simulink model "bh_dewarp_test"  (R2017a)
settings: Solver=FixedStepDiscrete  StartTime=0.0  StopTime=15  RelTol=1e-3
PreLoadFcn:
  | bh_create_cv_neareset_BUS_OBJ_for_simulink()
  | fprintf('\n\n### just did a preload TASK !');
undefined symbols (not defined in the file or in its folder): gray
libraries: dspvision x1, visiongeotforms x1
settings Model: FPTRunName=Active  ExtModeAutoUpdateStatusClock=off  Creator=The MathWorks, Inc.  LastModifiedBy=bhorton
settings DataIOCC: LimitDataPoints=on  SaveFormat=Array  SaveOutput=off  SaveTime=off  SignalLoggingName=sigsOut
settings OptimizationCC: ExpressionDepthLimit=2147483647  InitFltsAndDblsToZero=on  LifeSpan=inf  BufferReusableBoundary=off
settings DebuggingCC: SaveWithParameterizedLinksMsg=none  UnderspecifiedInitializationDetection=Classic  MergeDetectMultiDrivingBlocksExec=none  CheckExecutionContextPreStartOutputMsg=on  CheckExecutionContextRuntimeOutputMsg=on  SignalResolutionControl=TryResolveAllWithWarning  MultiTaskDSMMsg=warning  MultiTaskCondExecSysMsg=none  ParameterPrecisionLossMsg=none  FcnCallInpInsideContextMsg=warning  BusObjectLabelMismatch=none  StateNameClashWarn=warning  StrictBusMsg=None  SFUnexpectedBacktrackingDiag=warning  SFNoUnconditionalDefaultTransitionDiag=warning  SFExecutionAtInitializationDiag=none
settings HardwareCC: ProdBitPerPointer=32  ProdBitPerSizeT=32  ProdBitPerPtrDiffT=32  ProdLargestAtomicFloat=None  ProdIntDivRoundTo=Undefined  ProdEndianess=Unspecified  ProdWordSize=32  ProdHWDeviceType=32-bit Generic  TargetBitPerPointer=64  TargetBitPerSizeT=64  TargetBitPerPtrDiffT=64  TargetLongLongMode=on  TargetIntDivRoundTo=Zero  TargetEndianess=LittleEndian  TargetWordSize=64  TargetHWDeviceType=Generic->MATLAB Host Computer  ProdEqTarget=off
settings ModelReferenceCC: PropagateSignalLabelsOutOfModel=off
settings GRTTargetCC: TargetFcnLib=ansi_tfl_tmw.mat  TargetLangStandard=C89/C90 (ANSI)  GeneratePreprocessorConditionals=Disable all  CombineOutputUpdateFcns=off  GRTInterface=on
settings ConfigComp: CovMetricSettings=dw  CovHtmlReporting=on  CovSaveCumulativeToWorkspaceVar=on  CovSaveSingleToWorkspaceVar=on  CovExternalEMLEnable=off

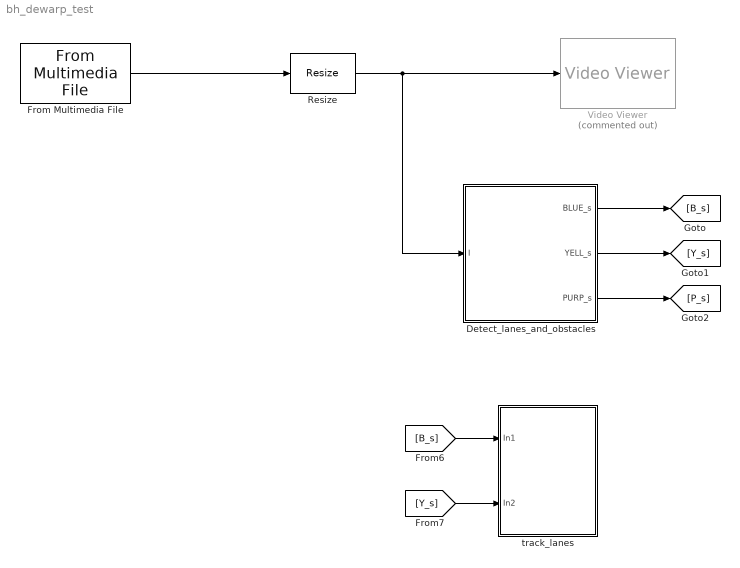
== system bh_dewarp_test ==
  Detect_lanes_and_obstacles : Subsystem
  From Multimedia File : dspvision/From Multimedia File  inputFilename=C:\bh\users_EV\Competitions\QUT_Droid_Racing_Challenge\DEMOS\sandpit\bh_vis_for_CODEGEN\TEST_VIDEO_FOR_SL_240x320.avi  loop=on  numPlays=1  outputStreams=Video only  videoDataType=uint8  audioDataType=int16  inheritSampleTime=on  userDefinedSampleTime=1/30  noAudioOutput=off  isIntensityVideo=off  fourcc=RGB  colorVideoFormat=One multidimensional signal  outputEOF=off  dataOrg=Column-major  audioFrameSize=1024  computeAudioFrameSize=off  outSamplingMode=Frame based
      settings: SourceProductBaseCode=VP
  Resize : visiongeotforms/Resize  specify=Number of output rows and columns  rfactor=[180 240]  outCols=25  outRows=25  outRowsCols=[180 240]  interp_method=Bilinear  antialias=off  useROI=off  roiFlag=off  prodOutputMode=Binary point scaling  prodOutputWordLength=32  prodOutputFracLength=10  roundingMode=Nearest  overflowMode=on
      settings: SourceProductName=Computer Vision System Toolbox  SourceProductBaseCode=VP
  Video Viewer : VideoViewer  Commented=on  colormapValue=gray(256)  FigPos=[2034 1219 418 304]
  track_lanes : Subsystem
  wires:
  From Multimedia File/1 -> Resize/1
  Detect_lanes_and_obstacles/1(BLUE_s) -> [B_s]
  Detect_lanes_and_obstacles/2(YELL_s) -> [Y_s]
  Detect_lanes_and_obstacles/3(PURP_s) -> [P_s]
  [B_s] -> track_lanes/1(In1)
  Resize/1 -> Detect_lanes_and_obstacles/1(I), Video Viewer/1
  [Y_s] -> track_lanes/2(In2)

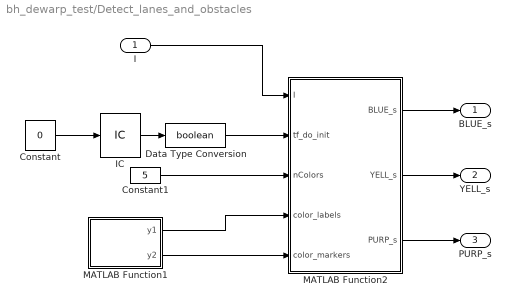
== system bh_dewarp_test/Detect_lanes_and_obstacles ==
  I : Inport
  Constant : Constant  Value=0  OutDataTypeStr=boolean
  Constant1 : Constant  Value=5  OutDataTypeStr=double
  Data Type Conversion : DataTypeConversion  OutDataTypeStr=boolean
  IC : InitialCondition
  MATLAB Function1 : MATLAB Function  TreatAsAtomicUnit=on
  MATLAB Function2 : MATLAB Function  TreatAsAtomicUnit=on
  BLUE_s : Outport
  YELL_s : Outport  Port=2
  PURP_s : Outport  Port=3
  wires:
  Constant/1 -> IC/1
  Data Type Conversion/1 -> MATLAB Function2/2(tf_do_init)
  IC/1 -> Data Type Conversion/1
  Constant1/1 -> MATLAB Function2/3(nColors)
  MATLAB Function1/1(y1) -> MATLAB Function2/4(color_labels)
  MATLAB Function1/2(y2) -> MATLAB Function2/5(color_markers)
  I/1 -> MATLAB Function2/1(I)
  MATLAB Function2/3(PURP_s) -> PURP_s/1
  MATLAB Function2/2(YELL_s) -> YELL_s/1
  MATLAB Function2/1(BLUE_s) -> BLUE_s/1

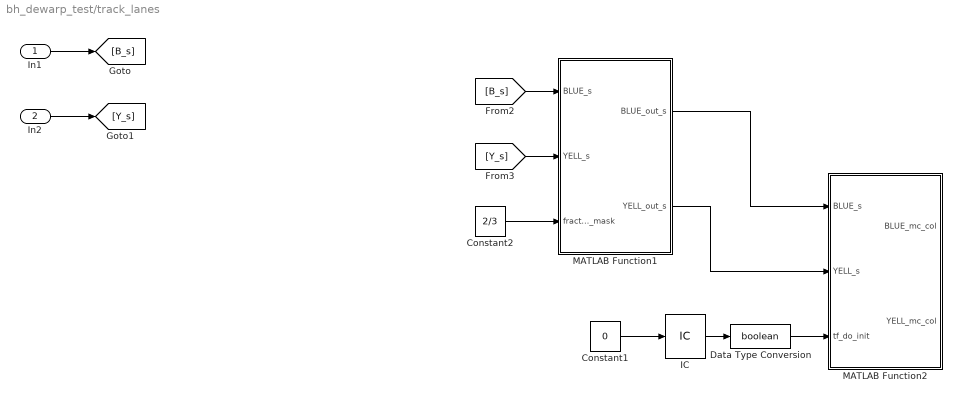
== system bh_dewarp_test/track_lanes ==
  In1 : Inport
  In2 : Inport  Port=2
  Constant1 : Constant  Value=0  OutDataTypeStr=boolean
  Constant2 : Constant  Value=2/3  OutDataTypeStr=double
  Data Type Conversion : DataTypeConversion  OutDataTypeStr=boolean
  IC : InitialCondition
  MATLAB Function1 : MATLAB Function  TreatAsAtomicUnit=on
  MATLAB Function2 : MATLAB Function  TreatAsAtomicUnit=on
  wires:
  In2/1 -> [Y_s]
  In1/1 -> [B_s]
  IC/1 -> Data Type Conversion/1
  Constant1/1 -> IC/1
  Data Type Conversion/1 -> MATLAB Function2/3(tf_do_init)
  MATLAB Function1/2(YELL_out_s) -> MATLAB Function2/2(YELL_s)
  MATLAB Function1/1(BLUE_out_s) -> MATLAB Function2/1(BLUE_s)
  [Y_s] -> MATLAB Function1/2(YELL_s)
  [B_s] -> MATLAB Function1/1(BLUE_s)
  Constant2/1 -> MATLAB Function1/3(fract_for_top_mask)

== matlab function bh_dewarp_test/Detect_lanes_and_obstacles/MATLAB Function1 ==
  data: y1 output; y2 output
function [y1, y2] = fcn()

y1 = [0,1,2,3,4];

y2 = [ ...
       -7.8436  -30.0394;
      -10.2908   36.4110;
       42.5297   -8.7231;
        2.1904    1.6907;
        4.0686    3.2113;
        ];
    
end

== matlab function bh_dewarp_test/track_lanes/MATLAB Function1 ==
  data: BLUE_s input Bus: lane_info_BUS; YELL_s input Bus: lane_info_BUS; fract_for_top_mask input; BLUE_out_s output Bus: lane_info_BUS; YELL_out_s output Bus: lane_info_BUS
function [BLUE_out_s, YELL_out_s] = ...
     pre_process_lanes(BLUE_s, YELL_s, fract_for_top_mask) %#codegen

coder.extrinsic('bh_my_lane_preprocess_mask')

[BLUE_out_s, YELL_out_s] = ...
    bh_my_lane_preprocess_mask(BLUE_s, YELL_s, fract_for_top_mask);


end

== matlab function bh_dewarp_test/Detect_lanes_and_obstacles/MATLAB Function2 ==
  data: I input; BLUE_s output Bus: lane_info_BUS; tf_do_init input; YELL_s output Bus: lane_info_BUS; PURP_s output Bus: box_info_BUS; nColors input; color_labels input; color_markers input
function [BLUE_s, YELL_s, PURP_s] = fcn(I, tf_do_init, ...
                                        nColors, color_labels, color_markers)

coder.extrinsic('bh_my_detect_ALGORITHM_for_codegen')

marker_s.nColors       = nColors;
marker_s.color_labels  = color_labels;
marker_s.color_markers = color_markers;

[BLUE_s, YELL_s, PURP_s] = bh_my_detect_ALGORITHM_for_codegen(I, tf_do_init, marker_s);

end

== matlab function bh_dewarp_test/track_lanes/MATLAB Function2 ==
  data: BLUE_s input Bus: lane_info_BUS; YELL_s input Bus: lane_info_BUS; BLUE_mc_col output double; tf_do_init input; YELL_mc_col output double
function [BLUE_mc_col, YELL_mc_col] = track_lanes(BLUE_s, YELL_s, tf_do_init) %#codegen

coder.extrinsic('bh_my_track_ALGORITHM_for_codegen')

BLUE_mc_col = [0;0];
YELL_mc_col = [0;0];

[BLUE_mc_col, YELL_mc_col]  = ...
    bh_my_track_ALGORITHM_for_codegen(BLUE_s, YELL_s, tf_do_init);

end
